simulink model "SimulinkAnalysisofCheetahTail"  (R2022a)
settings: Solver=FixedStepAuto  StartTime=0.0  StopTime=0.6  FixedStep=0.001  RelTol=1e-3
undefined symbols (not defined in the file): B_cg_H, B_con_H, B_con_L, bar_len, cd_table, Cf, cl_table, g, gear_ratio, int_point_bar, int_point_tail, ITail, M_add, M_cg_H, M_cg_L, M_cg_W, Mb, Mm, Mt, psi3, rho, T_cg_H, T_fur_gap, T_length, T_width_major, T_width_minor, th2_initial, torque_constant, uncertainty_Forces, uncertainty_Position, Vf, windspeed
(part 1 of 21)
settings Model: Creator=brigh_000  LastModifiedBy=bright
settings SolverCC: AlgebraicLoopSolver=TrustRegion  AutoInsertRateTranBlk=on
settings DebuggingCC: AlgebraicLoopMsg=none  UnconnectedInputMsg=warning  UnconnectedOutputMsg=warning  UnconnectedLineMsg=warning  SFMachineParentedDataDiag=warning
settings RTWCC: DLArmComputeVersion=19.05

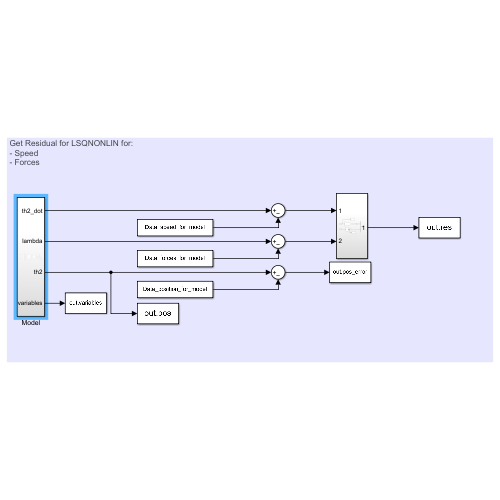
[thumbnail: Simulink's stored preview of the top-level diagram]
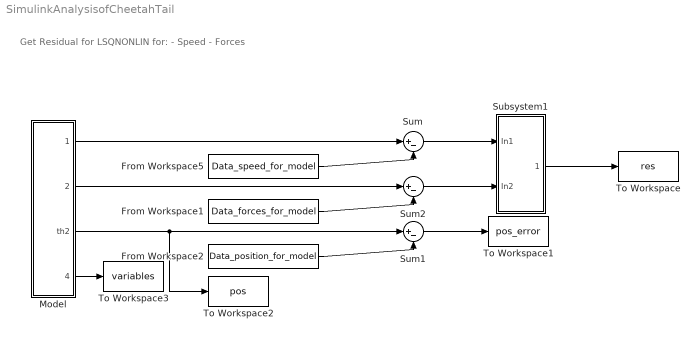
== system SimulinkAnalysisofCheetahTail ==
  note: Get Residual for LSQNONLIN for:
      | - Speed
      | - Forces
  From Workspace1 : FromWorkspace  VariableName=Data_forces_for_model  SampleTime=0.001  Interpolate=off  OutputAfterFinalValue=Holding final value
  From Workspace2 : FromWorkspace  VariableName=Data_position_for_model  SampleTime=0.001  Interpolate=off  OutputAfterFinalValue=Holding final value
  From Workspace5 : FromWorkspace  VariableName=Data_speed_for_model  SampleTime=0.001  Interpolate=off  OutputAfterFinalValue=Holding final value
  Model : Subsystem
  Subsystem1 : Subsystem
  Sum : Sum  Inputs=|+-
  Sum1 : Sum  Inputs=|+-
  Sum2 : Sum  Inputs=|+-
  To Workspace : ToWorkspace  VariableName=res  SampleTime=0.001
  To Workspace1 : ToWorkspace  VariableName=pos_error  SaveFormat=Timeseries  SampleTime=0.001
  To Workspace2 : ToWorkspace  VariableName=pos  SaveFormat=Timeseries  SampleTime=0.001
  To Workspace3 : ToWorkspace  VariableName=variables  SaveFormat=Timeseries  SampleTime=0.001
  wires:
  Sum/1 -> Subsystem1/1(In1)
  Model/3(th2) -> To Workspace2/1, Sum1/1
  Model/2(lambda) -> Sum2/1
  From Workspace1/1 -> Sum2/2
  Model/4(variables) -> To Workspace3/1
  From Workspace5/1 -> Sum/2
  Model/1(th2_dot) -> Sum/1
  Sum2/1 -> Subsystem1/2(In2)
  Subsystem1/1(Out1) -> To Workspace/1
  From Workspace2/1 -> Sum1/2
  Sum1/1 -> To Workspace1/1

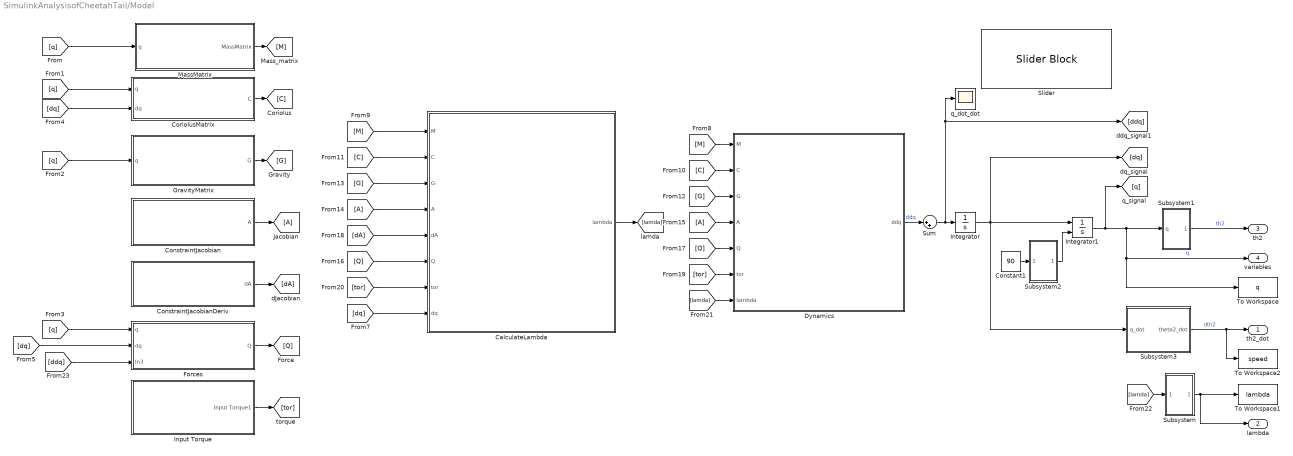
== system SimulinkAnalysisofCheetahTail/Model ==
  CalculateLambda : MATLAB Function  TreatAsAtomicUnit=on
  Constant1 : Constant  Value=90
  ConstraintJacobian : MATLAB Function  TreatAsAtomicUnit=on
  ConstraintJacobianDeriv : MATLAB Function  TreatAsAtomicUnit=on
  CoriolusMatrix : MATLAB Function  TreatAsAtomicUnit=on
  Dynamics : MATLAB Function  TreatAsAtomicUnit=on
  Forces : Subsystem
  From14 : From
  From15 : From
  GravityMatrix : MATLAB Function  TreatAsAtomicUnit=on
  Input Torque : Subsystem
  Integrator : Integrator  InitialCondition=[0;0;0;0;0;0;0;0]  ContinuousStateAttributes='velocity'
  Integrator1 : Integrator  InitialConditionSource=external  InitialCondition=[0;0;0;0;0;0;0*pi/180;0]  ContinuousStateAttributes='position'
  Jacobian : Goto
  MassMatrix : MATLAB Function  TreatAsAtomicUnit=on
  Slider : SliderBlock  LabelPosition=Bottom  ScaleMax=90  TickInterval=15
  Subsystem : Subsystem
  Subsystem1 : Subsystem
  Subsystem2 : Subsystem
  Subsystem3 : Subsystem
  Sum : Sum  Inputs=|++
  To Workspace : ToWorkspace  VariableName=q  SampleTime=0.001
  To Workspace1 : ToWorkspace  VariableName=lambda  SaveFormat=Timeseries  SampleTime=-1
  To Workspace2 : ToWorkspace  VariableName=speed  SaveFormat=Timeseries  SampleTime=0.001
  q_dot_dot : Scope
  th2_dot : Outport
  lambda : Outport  Port=2
  th2 : Outport  Port=3
  variables : Outport  Port=4
  wires:
  Subsystem/1(lambda) -> To Workspace1/1, lambda/1
  Subsystem1/1(theta2) -> th2/1  "th2"
  Subsystem2/1(Out1) -> Integrator1/2
  Constant1/1 -> Subsystem2/1(In1)
  Integrator/1 -> Subsystem3/1(q_dot), [dq], Integrator1/1
  Integrator1/1 -> [q], Subsystem1/1(q), To Workspace/1, variables/1  "q"
  Subsystem3/1(theta2_dot) -> To Workspace2/1, th2_dot/1  "dth2"
  [q] -> MassMatrix/1(q)
  [q] -> CoriolusMatrix/1(q)
  [q] -> GravityMatrix/1(q)
  [q] -> Forces/1(q)
  [dq] -> CoriolusMatrix/2(dq)
  [dq] -> Forces/2(dq)
  [dq] -> CalculateLambda/8(dq)
  MassMatrix/1(MassMatrix) -> [M]
  [M] -> Dynamics/1(M)
  [M] -> CalculateLambda/1(M)
  CoriolusMatrix/1(C) -> [C]
  [C] -> Dynamics/2(C)
  [C] -> CalculateLambda/2(C)
  ConstraintJacobianDeriv/1(dA) -> [dA]
  ConstraintJacobian/1(A) -> Jacobian/1
  GravityMatrix/1(G) -> [G]
  [G] -> CalculateLambda/3(G)
  [G] -> Dynamics/3(G)
  From14/1 -> CalculateLambda/4(A)
  From15/1 -> Dynamics/4(A)
  Forces/1(Q) -> [Q]
  [Q] -> CalculateLambda/6(Q)
  [Q] -> Dynamics/5(Q)
  [dA] -> CalculateLambda/5(dA)
  Input Torque/1(Input Torque1) -> [tor]
  [tor] -> Dynamics/6(tor)
  [tor] -> CalculateLambda/7(tor)
  CalculateLambda/1(lambda) -> [lamda]
  [lamda] -> Dynamics/7(lambda)
  [lamda] -> Subsystem/1(In1)
  Dynamics/1(ddq) -> Sum/1  "ddq"
  Sum/1 -> q_dot_dot/1, [ddq], Integrator/1
  [ddq] -> Forces/3(In3)

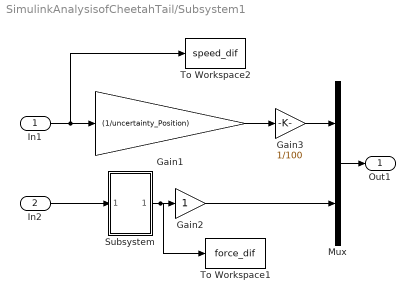
== system SimulinkAnalysisofCheetahTail/Subsystem1 ==
  In1 : Inport
  In2 : Inport  Port=2
  Gain1 : Gain  Gain=(1/uncertainty_Position)
  Gain2 : Gain
  Gain3 : Gain  Gain=1/100
  Mux : Mux  Inputs=2
  Subsystem : Subsystem
  To Workspace1 : ToWorkspace  VariableName=force_dif  SampleTime=0.001
  To Workspace2 : ToWorkspace  VariableName=speed_dif  SampleTime=0.001
  Out1 : Outport
  wires:
  In1/1 -> To Workspace2/1, Gain1/1
  Mux/1 -> Out1/1
  In2/1 -> Subsystem/1(In1)
  Subsystem/1(Out1) -> To Workspace1/1, Gain2/1
  Gain1/1 -> Gain3/1
  Gain2/1 -> Mux/2
  Gain3/1 -> Mux/1

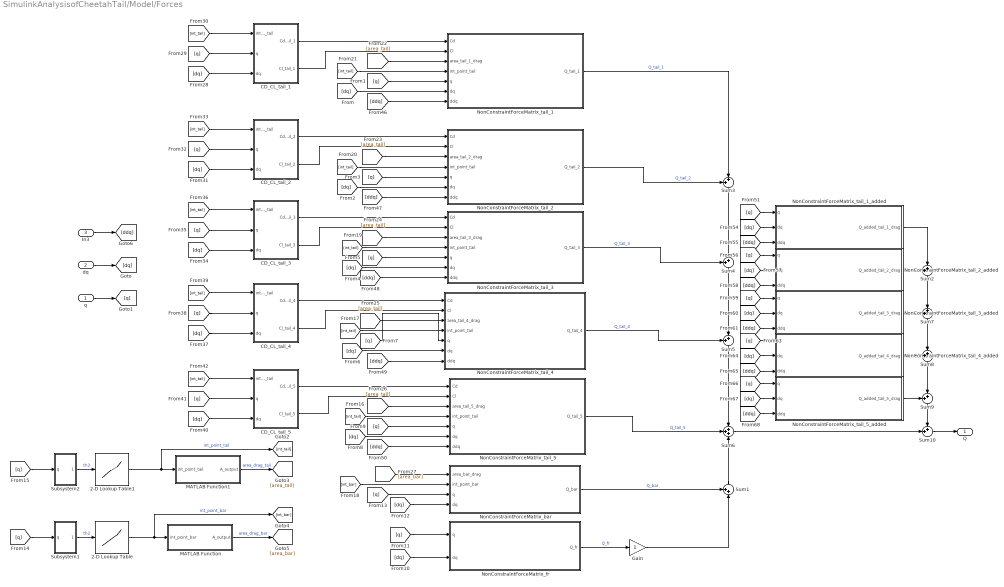
== system SimulinkAnalysisofCheetahTail/Model/Forces ==
  q : Inport
  dq : Inport  Port=2
  In3 : Inport  Port=3
  2-D Lookup Table : Lookup_n-D  NumberOfTableDimensions=1  LookupTableObject=bar_int_table  BreakpointsForDimension1=linspace(0,deg2rad(90),90)  BreakpointsForDimension2=[1:3]  Table=int_point_bar  InternalRulePriority=Speed  RndMeth=Simplest
  2-D Lookup Table1 : Lookup_n-D  NumberOfTableDimensions=1  LookupTableObject=bar_int_table  BreakpointsForDimension1=linspace(0,deg2rad(90),90)  BreakpointsForDimension2=[1:3]  Table=int_point_tail  InternalRulePriority=Speed  RndMeth=Simplest
  CD_CL_tail_1 : Subsystem
  CD_CL_tail_2 : Subsystem
  CD_CL_tail_3 : Subsystem
  CD_CL_tail_4 : Subsystem
  CD_CL_tail_5 : Subsystem
  Gain : Gain
  MATLAB Function : MATLAB Function  TreatAsAtomicUnit=on
  MATLAB Function1 : MATLAB Function  TreatAsAtomicUnit=on
  NonConstraintForceMatrix_bar : MATLAB Function  TreatAsAtomicUnit=on
  NonConstraintForceMatrix_fr : MATLAB Function  TreatAsAtomicUnit=on
  NonConstraintForceMatrix_tail_1 : MATLAB Function  TreatAsAtomicUnit=on
  NonConstraintForceMatrix_tail_1_added : MATLAB Function  TreatAsAtomicUnit=on
  NonConstraintForceMatrix_tail_2 : MATLAB Function  TreatAsAtomicUnit=on
  NonConstraintForceMatrix_tail_2_added : MATLAB Function  TreatAsAtomicUnit=on
  NonConstraintForceMatrix_tail_3 : MATLAB Function  TreatAsAtomicUnit=on
  NonConstraintForceMatrix_tail_3_added : MATLAB Function  TreatAsAtomicUnit=on
  NonConstraintForceMatrix_tail_4 : MATLAB Function  TreatAsAtomicUnit=on
  NonConstraintForceMatrix_tail_4_added : MATLAB Function  TreatAsAtomicUnit=on
  NonConstraintForceMatrix_tail_5 : MATLAB Function  TreatAsAtomicUnit=on
  NonConstraintForceMatrix_tail_5_added : MATLAB Function  TreatAsAtomicUnit=on
  Subsystem1 : Subsystem
  Subsystem2 : Subsystem
  Sum{1..5,7..10} (9 alike) : Sum  Inputs=++|
  Sum6 : Sum  Inputs=+++
  Q : Outport
  wires:
  NonConstraintForceMatrix_tail_4/1(Q_tail_4) -> Sum5/1  "Q_tail_4"
  NonConstraintForceMatrix_tail_5/1(Q_tail_5) -> Sum6/2  "Q_tail_5"
  NonConstraintForceMatrix_fr/1(Q_fr) -> Gain/1  "Q_fr"
  NonConstraintForceMatrix_bar/1(Q_bar) -> Sum1/1  "Q_bar"
  NonConstraintForceMatrix_tail_3/1(Q_tail_3) -> Sum4/1  "Q_tail_3"
  Sum1/1 -> Sum6/3
  dq/1 -> [dq]
  q/1 -> [q]
  [dq] -> NonConstraintForceMatrix_tail_1/6(dq)
  [dq] -> NonConstraintForceMatrix_tail_2/6(dq)
  [q] -> NonConstraintForceMatrix_tail_2/5(q)
  [q] -> NonConstraintForceMatrix_tail_3/5(q)
  [dq] -> NonConstraintForceMatrix_tail_3/6(dq)
  [q] -> NonConstraintForceMatrix_tail_4/5(q)
  [dq] -> NonConstraintForceMatrix_tail_4/6(dq)
  [dq] -> NonConstraintForceMatrix_tail_5/6(dq)
  [q] -> NonConstraintForceMatrix_fr/1(q)
  [dq] -> NonConstraintForceMatrix_bar/4(dq)
  Sum3/1 -> Sum4/2
  Sum4/1 -> Sum5/2
  NonConstraintForceMatrix_tail_1/1(Q_tail_1) -> Sum3/2  "Q_tail_1"
  NonConstraintForceMatrix_tail_2/1(Q_tail_2) -> Sum3/1  "Q_tail_2"
  Sum5/1 -> Sum6/1
  [dq] -> NonConstraintForceMatrix_fr/2(dq)
  Gain/1 -> Sum1/2
  [q] -> NonConstraintForceMatrix_tail_1/5(q)
  [q] -> NonConstraintForceMatrix_tail_5/5(q)
  2-D Lookup Table/1 -> [int_bar], MATLAB Function/1(int_point_bar)  "int_point_bar"
  Subsystem1/1(theta2) -> 2-D Lookup Table/1  "th2"
  Subsystem2/1(theta2) -> 2-D Lookup Table1/1  "th2"
  2-D Lookup Table1/1 -> [int_tail], MATLAB Function1/1(int_point_tail)  "int_point_tail"
  [q] -> Subsystem2/1(q)
  MATLAB Function/1(A_output) -> [area_bar]  "area_drag_bar"
  MATLAB Function1/1(A_output) -> [area_tail]  "area_drag_tail"
  [q] -> Subsystem1/1(q)
  [q] -> NonConstraintForceMatrix_bar/3(q)
  [int_tail] -> NonConstraintForceMatrix_tail_5/4(int_point_tail)
  [int_tail] -> NonConstraintForceMatrix_tail_4/4(int_point_tail)
  [int_tail] -> NonConstraintForceMatrix_tail_3/4(int_point_tail)
  [int_tail] -> NonConstraintForceMatrix_tail_2/4(int_point_tail)
  [int_tail] -> NonConstraintForceMatrix_tail_1/4(int_point_tail)
  [area_tail] -> NonConstraintForceMatrix_tail_1/3(area_tail_1_drag)
  [area_tail] -> NonConstraintForceMatrix_tail_2/3(area_tail_2_drag)
  [area_tail] -> NonConstraintForceMatrix_tail_3/3(area_tail_3_drag)
  [area_tail] -> NonConstraintForceMatrix_tail_4/3(area_tail_4_drag)
  [area_tail] -> NonConstraintForceMatrix_tail_5/3(area_tail_5_drag)
  [area_bar] -> NonConstraintForceMatrix_bar/1(area_bar_drag)
  [int_bar] -> NonConstraintForceMatrix_bar/2(int_point_bar)
  [dq] -> CD_CL_tail_1/3(dq)
  [q] -> CD_CL_tail_1/2(q)
  [int_tail] -> CD_CL_tail_1/1(int_point_tail)
  [dq] -> CD_CL_tail_2/3(dq)
  [int_tail] -> CD_CL_tail_2/1(int_point_tail)
  [q] -> CD_CL_tail_2/2(q)
  [dq] -> CD_CL_tail_3/3(dq)
  [int_tail] -> CD_CL_tail_3/1(int_point_tail)
  [q] -> CD_CL_tail_3/2(q)
  [dq] -> CD_CL_tail_4/3(dq)
  [int_tail] -> CD_CL_tail_4/1(int_point_tail)
  [q] -> CD_CL_tail_4/2(q)
  [dq] -> CD_CL_tail_5/3(dq)
  [int_tail] -> CD_CL_tail_5/1(int_point_tail)
  [q] -> CD_CL_tail_5/2(q)
  CD_CL_tail_1/1(Cd_tail_1) -> NonConstraintForceMatrix_tail_1/1(Cd)
  CD_CL_tail_1/2(Cl_tail_1) -> NonConstraintForceMatrix_tail_1/2(Cl)
  CD_CL_tail_2/1(Cd_tail_2) -> NonConstraintForceMatrix_tail_2/1(Cd)
  CD_CL_tail_2/2(Cl_tail_2) -> NonConstraintForceMatrix_tail_2/2(Cl)
  CD_CL_tail_4/1(Cd_tail_4) -> NonConstraintForceMatrix_tail_4/1(Cd)
  CD_CL_tail_4/2(Cl_tail_4) -> NonConstraintForceMatrix_tail_4/2(Cl)
  CD_CL_tail_5/1(Cd_tail_5) -> NonConstraintForceMatrix_tail_5/1(Cd)
  CD_CL_tail_5/2(Cl_tail_5) -> NonConstraintForceMatrix_tail_5/2(Cl)
  In3/1 -> [ddq]
  [ddq] -> NonConstraintForceMatrix_tail_1/7(ddq)
  [ddq] -> NonConstraintForceMatrix_tail_2/7(ddq)
  [ddq] -> NonConstraintForceMatrix_tail_3/7(ddq)
  [ddq] -> NonConstraintForceMatrix_tail_4/7(ddq)
  [ddq] -> NonConstraintForceMatrix_tail_5/7(ddq)
  NonConstraintForceMatrix_tail_4_added/1(Q_added_tail_4_drag) -> Sum8/1
  NonConstraintForceMatrix_tail_5_added/1(Q_added_tail_5_drag) -> Sum9/1
  Sum8/1 -> Sum9/2
  Sum7/1 -> Sum8/2
  NonConstraintForceMatrix_tail_3_added/1(Q_added_tail_3_drag) -> Sum7/1
  Sum2/1 -> Sum7/2
  NonConstraintForceMatrix_tail_2_added/1(Q_added_tail_2_drag) -> Sum2/1
  NonConstraintForceMatrix_tail_1_added/1(Q_added_tail_1_drag) -> Sum2/2
  Sum9/1 -> Sum10/1
  Sum6/1 -> Sum10/2
  Sum10/1 -> Q/1
  [q] -> NonConstraintForceMatrix_tail_1_added/1(q)
  [dq] -> NonConstraintForceMatrix_tail_1_added/2(dq)
  [ddq] -> NonConstraintForceMatrix_tail_1_added/3(ddq)
  [ddq] -> NonConstraintForceMatrix_tail_2_added/3(ddq)
  [dq] -> NonConstraintForceMatrix_tail_2_added/2(dq)
  [q] -> NonConstraintForceMatrix_tail_2_added/1(q)
  [q] -> NonConstraintForceMatrix_tail_3_added/1(q)
  [dq] -> NonConstraintForceMatrix_tail_3_added/2(dq)
  [ddq] -> NonConstraintForceMatrix_tail_3_added/3(ddq)
  [ddq] -> NonConstraintForceMatrix_tail_4_added/3(ddq)
  [dq] -> NonConstraintForceMatrix_tail_4_added/2(dq)
  [q] -> NonConstraintForceMatrix_tail_4_added/1(q)
  [q] -> NonConstraintForceMatrix_tail_5_added/1(q)
  [dq] -> NonConstraintForceMatrix_tail_5_added/2(dq)
  [ddq] -> NonConstraintForceMatrix_tail_5_added/3(ddq)
  CD_CL_tail_3/1(Cd_tail_3) -> NonConstraintForceMatrix_tail_3/1(Cd)
  CD_CL_tail_3/2(Cl_tail_3) -> NonConstraintForceMatrix_tail_3/2(Cl)

== system SimulinkAnalysisofCheetahTail/Model/Input Torque ==
  From Workspace3 : FromWorkspace  VariableName=Data_current_for_model  SampleTime=0.001
  Gear Ratio1 : Gain  Gain=gear_ratio
  Motor Efficiency1 : Gain
  Torque Constant1 : Gain  Gain=(torque_constant/1000)
  Input Torque1 : Outport
  wires:
  Gear Ratio1/1 -> Motor Efficiency1/1  "Tail_torque"
  Motor Efficiency1/1 -> Input Torque1/1  "Tail_torque_final"
  Torque Constant1/1 -> Gear Ratio1/1  "Motor_torque"
  From Workspace3/1 -> Torque Constant1/1  "Measured_current"

== system SimulinkAnalysisofCheetahTail/Model/Subsystem ==
  In1 : Inport
  Demux1 : Demux  Outputs=7
  Mux : Mux  Inputs=6
  Terminator : Terminator
  lambda : Outport
  wires:
  Demux1/3 -> Mux/3
  Demux1/4 -> Mux/4
  Demux1/1 -> Mux/1
  Demux1/6 -> Mux/6
  Demux1/5 -> Mux/5
  Demux1/7 -> Terminator/1
  Demux1/2 -> Mux/2
  In1/1 -> Demux1/1
  Mux/1 -> lambda/1

== system SimulinkAnalysisofCheetahTail/Model/Subsystem1 ==
  q : Inport
  Demux : Demux  Outputs=8
  Mux : Mux  Inputs=7
  Terminator1 : Terminator
  theta2 : Outport
  wires:
  Demux/7 -> theta2/1
  Demux/5 -> Mux/5
  Demux/1 -> Mux/1
  Demux/8 -> Mux/7
  Mux/1 -> Terminator1/1
  Demux/2 -> Mux/2
  Demux/4 -> Mux/4
  Demux/6 -> Mux/6
  Demux/3 -> Mux/3
  q/1 -> Demux/1

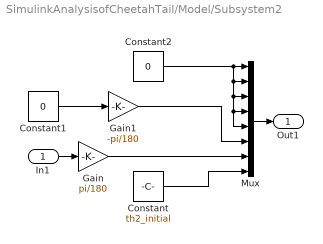
== system SimulinkAnalysisofCheetahTail/Model/Subsystem2 ==
  In1 : Inport
  Constant : Constant  Value=th2_initial  SampleTime=0.001
  Constant1 : Constant  Value=0  SampleTime=0.001
  Constant2 : Constant  Value=0  SampleTime=0.001
  Gain : Gain  Gain=pi/180
  Gain1 : Gain  Gain=-pi/180
  Mux : Mux  Inputs=8
  Out1 : Outport
  wires:
  In1/1 -> Gain/1
  Constant2/1 -> Mux/5, Mux/4, Mux/3, Mux/2, Mux/1
  Gain/1 -> Mux/7
  Constant/1 -> Mux/8
  Mux/1 -> Out1/1
  Constant1/1 -> Gain1/1
  Gain1/1 -> Mux/6

== system SimulinkAnalysisofCheetahTail/Model/Subsystem3 ==
  q_dot : Inport
  Demux : Demux  Outputs=8
  Mux : Mux  Inputs=7
  Terminator1 : Terminator
  theta2_dot : Outport
  wires:
  Demux/7 -> theta2_dot/1
  Demux/5 -> Mux/5
  Demux/1 -> Mux/1
  Demux/8 -> Mux/7
  Mux/1 -> Terminator1/1
  Demux/2 -> Mux/2
  Demux/4 -> Mux/4
  Demux/6 -> Mux/6
  Demux/3 -> Mux/3
  q_dot/1 -> Demux/1

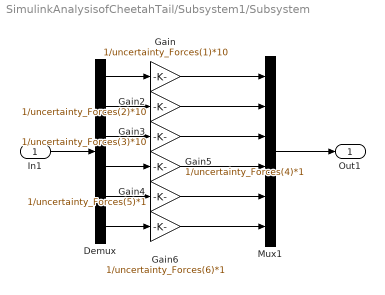
== system SimulinkAnalysisofCheetahTail/Subsystem1/Subsystem ==
  In1 : Inport
  Demux : Demux  Outputs=6
  Gain : Gain  Gain=1/uncertainty_Forces(1)*10
  Gain2 : Gain  Gain=1/uncertainty_Forces(2)*10
  Gain3 : Gain  Gain=1/uncertainty_Forces(3)*10
  Gain4 : Gain  Gain=1/uncertainty_Forces(5)*1
  Gain5 : Gain  Gain=1/uncertainty_Forces(4)*1
  Gain6 : Gain  Gain=1/uncertainty_Forces(6)*1
  Mux1 : Mux  Inputs=6
  Out1 : Outport
  wires:
  Gain6/1 -> Mux1/6
  Demux/1 -> Gain/1
  Gain/1 -> Mux1/1
  Gain5/1 -> Mux1/4
  Gain2/1 -> Mux1/2
  Gain3/1 -> Mux1/3
  Demux/2 -> Gain2/1
  Mux1/1 -> Out1/1
  Gain4/1 -> Mux1/5
  In1/1 -> Demux/1
  Demux/6 -> Gain6/1
  Demux/5 -> Gain4/1
  Demux/4 -> Gain5/1
  Demux/3 -> Gain3/1

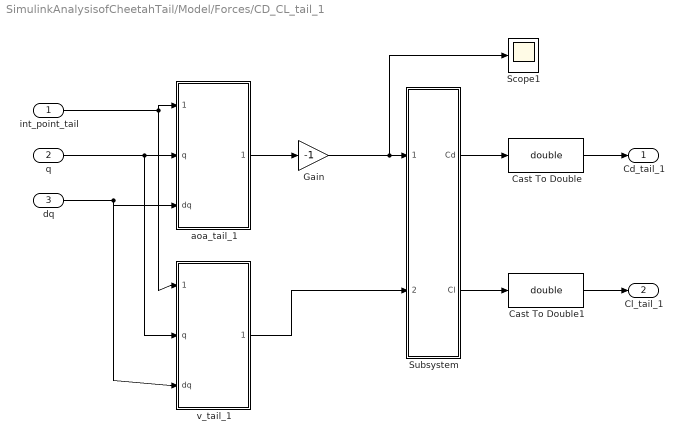
== system SimulinkAnalysisofCheetahTail/Model/Forces/CD_CL_tail_1 ==
  int_point_tail : Inport
  q : Inport  Port=2
  dq : Inport  Port=3
  Cast To Double : DataTypeConversion  OutDataTypeStr=double  SaturateOnIntegerOverflow=off  RndMeth=Floor
  Cast To Double1 : DataTypeConversion  OutDataTypeStr=double  SaturateOnIntegerOverflow=off  RndMeth=Floor
  Gain : Gain  Gain=-1
  Scope1 : Scope
  Subsystem : Subsystem
  aoa_tail_1 : MATLAB Function  TreatAsAtomicUnit=on
  v_tail_1 : MATLAB Function  TreatAsAtomicUnit=on
  Cd_tail_1 : Outport
  Cl_tail_1 : Outport  Port=2
  wires:
  q/1 -> v_tail_1/2(q), aoa_tail_1/2(q)
  int_point_tail/1 -> v_tail_1/1(int_point_tail), aoa_tail_1/1(int_point_tail)
  dq/1 -> v_tail_1/3(dq), aoa_tail_1/3(dq)
  Subsystem/2(Cl) -> Cast To Double1/1
  aoa_tail_1/1(aoa_tail_1) -> Gain/1
  Subsystem/1(Cd) -> Cast To Double/1
  v_tail_1/1(v_tail_1_speed) -> Subsystem/2(Velocity)
  Cast To Double/1 -> Cd_tail_1/1
  Cast To Double1/1 -> Cl_tail_1/1
  Gain/1 -> Scope1/1, Subsystem/1(Angles)

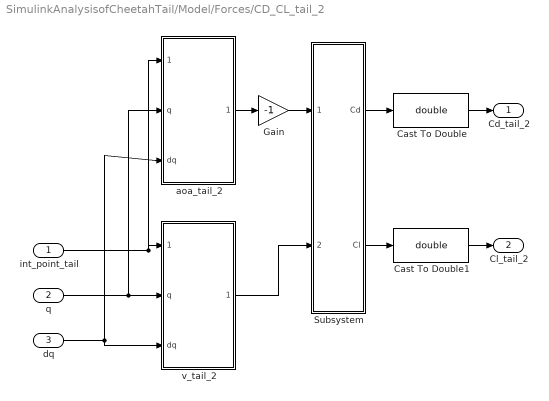
== system SimulinkAnalysisofCheetahTail/Model/Forces/CD_CL_tail_2 ==
  int_point_tail : Inport
  q : Inport  Port=2
  dq : Inport  Port=3
  Cast To Double : DataTypeConversion  OutDataTypeStr=double  SaturateOnIntegerOverflow=off  RndMeth=Floor
  Cast To Double1 : DataTypeConversion  OutDataTypeStr=double  SaturateOnIntegerOverflow=off  RndMeth=Floor
  Gain : Gain  Gain=-1
  Subsystem : Subsystem
  aoa_tail_2 : MATLAB Function  TreatAsAtomicUnit=on
  v_tail_2 : MATLAB Function  TreatAsAtomicUnit=on
  Cd_tail_2 : Outport
  Cl_tail_2 : Outport  Port=2
  wires:
  dq/1 -> v_tail_2/3(dq), aoa_tail_2/3(dq)
  q/1 -> aoa_tail_2/2(q), v_tail_2/2(q)
  int_point_tail/1 -> aoa_tail_2/1(int_point_tail), v_tail_2/1(int_point_tail)
  Subsystem/2(Cl) -> Cast To Double1/1
  aoa_tail_2/1(aoa_tail_2) -> Gain/1
  Subsystem/1(Cd) -> Cast To Double/1
  v_tail_2/1(v_tail_2_speed) -> Subsystem/2(Velocity)
  Cast To Double/1 -> Cd_tail_2/1
  Cast To Double1/1 -> Cl_tail_2/1
  Gain/1 -> Subsystem/1(Angles)

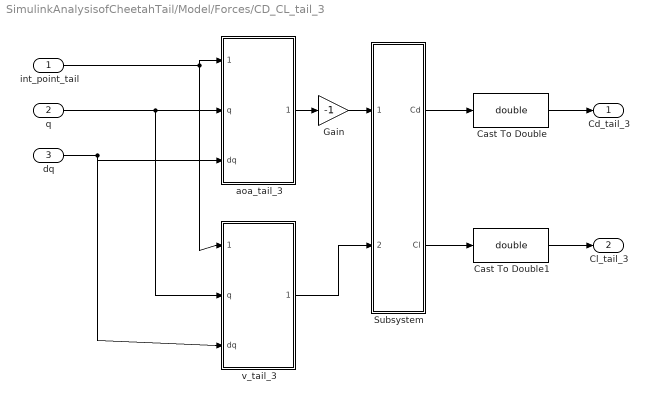
== system SimulinkAnalysisofCheetahTail/Model/Forces/CD_CL_tail_3 ==
  int_point_tail : Inport
  q : Inport  Port=2
  dq : Inport  Port=3
  Cast To Double : DataTypeConversion  OutDataTypeStr=double  SaturateOnIntegerOverflow=off  RndMeth=Floor
  Cast To Double1 : DataTypeConversion  OutDataTypeStr=double  SaturateOnIntegerOverflow=off  RndMeth=Floor
  Gain : Gain  Gain=-1
  Subsystem : Subsystem
  aoa_tail_3 : MATLAB Function  TreatAsAtomicUnit=on
  v_tail_3 : MATLAB Function  TreatAsAtomicUnit=on
  Cd_tail_3 : Outport
  Cl_tail_3 : Outport  Port=2
  wires:
  int_point_tail/1 -> v_tail_3/1(int_point_tail), aoa_tail_3/1(int_point_tail)
  q/1 -> v_tail_3/2(q), aoa_tail_3/2(q)
  dq/1 -> aoa_tail_3/3(dq), v_tail_3/3(dq)
  Subsystem/1(Cd) -> Cast To Double/1
  Subsystem/2(Cl) -> Cast To Double1/1
  aoa_tail_3/1(aoa_tail_3) -> Gain/1
  v_tail_3/1(v_tail_3_speed) -> Subsystem/2(Velocity)
  Cast To Double/1 -> Cd_tail_3/1
  Cast To Double1/1 -> Cl_tail_3/1
  Gain/1 -> Subsystem/1(Angles)

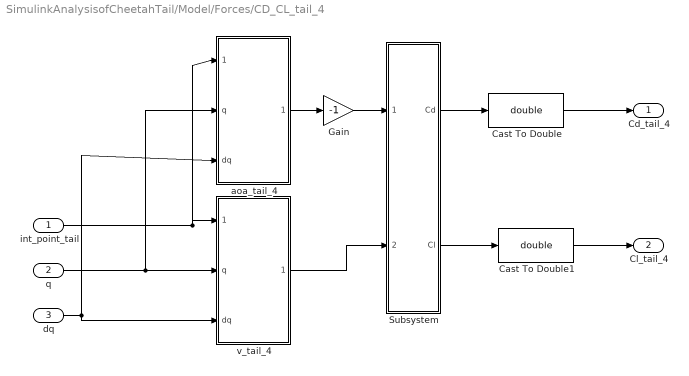
== system SimulinkAnalysisofCheetahTail/Model/Forces/CD_CL_tail_4 ==
  int_point_tail : Inport
  q : Inport  Port=2
  dq : Inport  Port=3
  Cast To Double : DataTypeConversion  OutDataTypeStr=double  SaturateOnIntegerOverflow=off  RndMeth=Floor
  Cast To Double1 : DataTypeConversion  OutDataTypeStr=double  SaturateOnIntegerOverflow=off  RndMeth=Floor
  Gain : Gain  Gain=-1
  Subsystem : Subsystem
  aoa_tail_4 : MATLAB Function  TreatAsAtomicUnit=on
  v_tail_4 : MATLAB Function  TreatAsAtomicUnit=on
  Cd_tail_4 : Outport
  Cl_tail_4 : Outport  Port=2
  wires:
  dq/1 -> aoa_tail_4/3(dq), v_tail_4/3(dq)
  int_point_tail/1 -> aoa_tail_4/1(int_point_tail), v_tail_4/1(int_point_tail)
  q/1 -> aoa_tail_4/2(q), v_tail_4/2(q)
  aoa_tail_4/1(aoa_tail_4) -> Gain/1
  v_tail_4/1(v_tail_4_speed) -> Subsystem/2(Velocity)
  Subsystem/1(Cd) -> Cast To Double/1
  Subsystem/2(Cl) -> Cast To Double1/1
  Cast To Double/1 -> Cd_tail_4/1
  Cast To Double1/1 -> Cl_tail_4/1
  Gain/1 -> Subsystem/1(Angles)

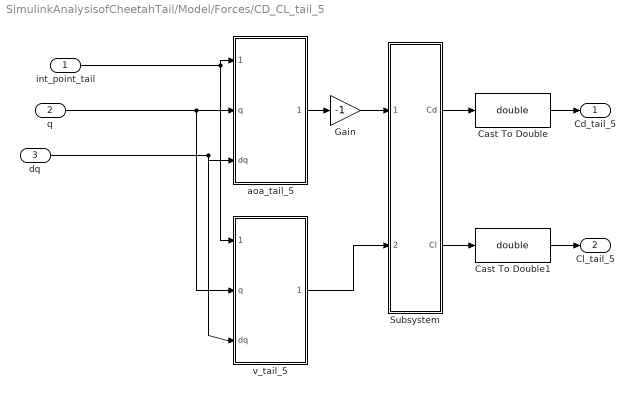
== system SimulinkAnalysisofCheetahTail/Model/Forces/CD_CL_tail_5 ==
  int_point_tail : Inport
  q : Inport  Port=2
  dq : Inport  Port=3
  Cast To Double : DataTypeConversion  OutDataTypeStr=double  SaturateOnIntegerOverflow=off  RndMeth=Floor
  Cast To Double1 : DataTypeConversion  OutDataTypeStr=double  SaturateOnIntegerOverflow=off  RndMeth=Floor
  Gain : Gain  Gain=-1
  Subsystem : Subsystem
  aoa_tail_5 : MATLAB Function  TreatAsAtomicUnit=on
  v_tail_5 : MATLAB Function  TreatAsAtomicUnit=on
  Cd_tail_5 : Outport
  Cl_tail_5 : Outport  Port=2
  wires:
  q/1 -> aoa_tail_5/2(q), v_tail_5/2(q)
  int_point_tail/1 -> v_tail_5/1(int_point_tail), aoa_tail_5/1(int_point_tail)
  dq/1 -> aoa_tail_5/3(dq), v_tail_5/3(dq)
  v_tail_5/1(v_tail_5_speed) -> Subsystem/2(Velocity)
  aoa_tail_5/1(aoa_tail_5) -> Gain/1
  Subsystem/1(Cd) -> Cast To Double/1
  Subsystem/2(Cl) -> Cast To Double1/1
  Cast To Double/1 -> Cd_tail_5/1
  Cast To Double1/1 -> Cl_tail_5/1
  Gain/1 -> Subsystem/1(Angles)

== system SimulinkAnalysisofCheetahTail/Model/Forces/Subsystem1 ==
  q : Inport
  Demux : Demux  Outputs=8
  Mux : Mux  Inputs=7
  Terminator1 : Terminator
  theta2 : Outport
  wires:
  Demux/7 -> theta2/1
  Demux/5 -> Mux/5
  Demux/1 -> Mux/1
  Demux/8 -> Mux/7
  Mux/1 -> Terminator1/1
  Demux/2 -> Mux/2
  Demux/4 -> Mux/4
  Demux/6 -> Mux/6
  Demux/3 -> Mux/3
  q/1 -> Demux/1

== system SimulinkAnalysisofCheetahTail/Model/Forces/Subsystem2 ==
  q : Inport
  Demux : Demux  Outputs=8
  Mux : Mux  Inputs=7
  Terminator1 : Terminator
  theta2 : Outport
  wires:
  Demux/7 -> theta2/1
  Demux/5 -> Mux/5
  Demux/1 -> Mux/1
  Demux/8 -> Mux/7
  Mux/1 -> Terminator1/1
  Demux/2 -> Mux/2
  Demux/4 -> Mux/4
  Demux/6 -> Mux/6
  Demux/3 -> Mux/3
  q/1 -> Demux/1

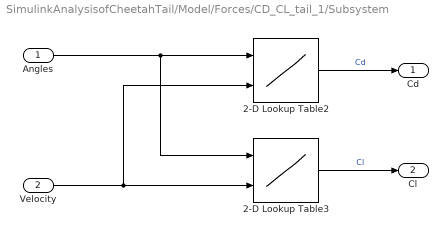
== system SimulinkAnalysisofCheetahTail/Model/Forces/CD_CL_tail_1/Subsystem ==
  Angles : Inport
  Velocity : Inport  Port=2
  2-D Lookup Table2 : Lookup_n-D  LookupTableObject=bar_int_table  BreakpointsForDimension1=deg2rad([0 15 30 45 60 75])  BreakpointsForDimension2=[10 20 30]  Table=cd_table  InternalRulePriority=Speed  RndMeth=Simplest
      settings: InputPortMap=u0,u1
  2-D Lookup Table3 : Lookup_n-D  LookupTableObject=bar_int_table  BreakpointsForDimension1=deg2rad([0 15 30 45 60 75])  BreakpointsForDimension2=[10 20 30]  Table=cl_table  InternalRulePriority=Speed  RndMeth=Simplest
      settings: InputPortMap=u0,u1
  Cd : Outport
  Cl : Outport  Port=2
  wires:
  Velocity/1 -> 2-D Lookup Table3/2, 2-D Lookup Table2/2
  Angles/1 -> 2-D Lookup Table2/1, 2-D Lookup Table3/1
  2-D Lookup Table2/1 -> Cd/1  "Cd"
  2-D Lookup Table3/1 -> Cl/1  "Cl"

== system SimulinkAnalysisofCheetahTail/Model/Forces/CD_CL_tail_2/Subsystem ==
  Angles : Inport
  Velocity : Inport  Port=2
  2-D Lookup Table2 : Lookup_n-D  LookupTableObject=bar_int_table  BreakpointsForDimension1=deg2rad([0 15 30 45 60 75])  BreakpointsForDimension2=[10 20 30]  Table=cd_table  InternalRulePriority=Speed  RndMeth=Simplest
      settings: InputPortMap=u0,u1
  2-D Lookup Table3 : Lookup_n-D  LookupTableObject=bar_int_table  BreakpointsForDimension1=deg2rad([0 15 30 45 60 75])  BreakpointsForDimension2=[10 20 30]  Table=cl_table  InternalRulePriority=Speed  RndMeth=Simplest
      settings: InputPortMap=u0,u1
  Cd : Outport
  Cl : Outport  Port=2
  wires:
  Velocity/1 -> 2-D Lookup Table3/2, 2-D Lookup Table2/2
  Angles/1 -> 2-D Lookup Table2/1, 2-D Lookup Table3/1
  2-D Lookup Table2/1 -> Cd/1  "Cd"
  2-D Lookup Table3/1 -> Cl/1  "Cl"

== system SimulinkAnalysisofCheetahTail/Model/Forces/CD_CL_tail_3/Subsystem ==
  Angles : Inport
  Velocity : Inport  Port=2
  2-D Lookup Table2 : Lookup_n-D  LookupTableObject=bar_int_table  BreakpointsForDimension1=deg2rad([0 15 30 45 60 75])  BreakpointsForDimension2=[10 20 30]  Table=cd_table  InternalRulePriority=Speed  RndMeth=Simplest
      settings: InputPortMap=u0,u1
  2-D Lookup Table3 : Lookup_n-D  LookupTableObject=bar_int_table  BreakpointsForDimension1=deg2rad([0 15 30 45 60 75])  BreakpointsForDimension2=[10 20 30]  Table=cl_table  InternalRulePriority=Speed  RndMeth=Simplest
      settings: InputPortMap=u0,u1
  Cd : Outport
  Cl : Outport  Port=2
  wires:
  Velocity/1 -> 2-D Lookup Table3/2, 2-D Lookup Table2/2
  Angles/1 -> 2-D Lookup Table2/1, 2-D Lookup Table3/1
  2-D Lookup Table2/1 -> Cd/1  "Cd"
  2-D Lookup Table3/1 -> Cl/1  "Cl"

== system SimulinkAnalysisofCheetahTail/Model/Forces/CD_CL_tail_4/Subsystem ==
  Angles : Inport
  Velocity : Inport  Port=2
  2-D Lookup Table2 : Lookup_n-D  LookupTableObject=bar_int_table  BreakpointsForDimension1=deg2rad([0 15 30 45 60 75])  BreakpointsForDimension2=[10 20 30]  Table=cd_table  InternalRulePriority=Speed  RndMeth=Simplest
      settings: InputPortMap=u0,u1
  2-D Lookup Table3 : Lookup_n-D  LookupTableObject=bar_int_table  BreakpointsForDimension1=deg2rad([0 15 30 45 60 75])  BreakpointsForDimension2=[10 20 30]  Table=cl_table  InternalRulePriority=Speed  RndMeth=Simplest
      settings: InputPortMap=u0,u1
  Cd : Outport
  Cl : Outport  Port=2
  wires:
  Velocity/1 -> 2-D Lookup Table3/2, 2-D Lookup Table2/2
  Angles/1 -> 2-D Lookup Table2/1, 2-D Lookup Table3/1
  2-D Lookup Table2/1 -> Cd/1  "Cd"
  2-D Lookup Table3/1 -> Cl/1  "Cl"

== system SimulinkAnalysisofCheetahTail/Model/Forces/CD_CL_tail_5/Subsystem ==
  Angles : Inport
  Velocity : Inport  Port=2
  2-D Lookup Table2 : Lookup_n-D  LookupTableObject=bar_int_table  BreakpointsForDimension1=deg2rad([0 15 30 45 60 75])  BreakpointsForDimension2=[10 20 30]  Table=cd_table  InternalRulePriority=Speed  RndMeth=Simplest
      settings: InputPortMap=u0,u1
  2-D Lookup Table3 : Lookup_n-D  LookupTableObject=bar_int_table  BreakpointsForDimension1=deg2rad([0 15 30 45 60 75])  BreakpointsForDimension2=[10 20 30]  Table=cl_table  InternalRulePriority=Speed  RndMeth=Simplest
      settings: InputPortMap=u0,u1
  Cd : Outport
  Cl : Outport  Port=2
  wires:
  Velocity/1 -> 2-D Lookup Table3/2, 2-D Lookup Table2/2
  Angles/1 -> 2-D Lookup Table2/1, 2-D Lookup Table3/1
  2-D Lookup Table2/1 -> Cd/1  "Cd"
  2-D Lookup Table3/1 -> Cl/1  "Cl"
